simulink subsystem "LuT"  (R2019b)
settings: Solver=VariableStepAuto  StartTime=0.0  StopTime=10.0  RelTol=1e-3
undefined symbols (not defined in the file or in its folder): C1_lut, C2_lut, OCV_lut, R0_est, R0_lut, R1_lut, R2_lut
settings Model: Creator=PcElettronicaDynamis  LastModifiedBy=PcElettronicaDynamis

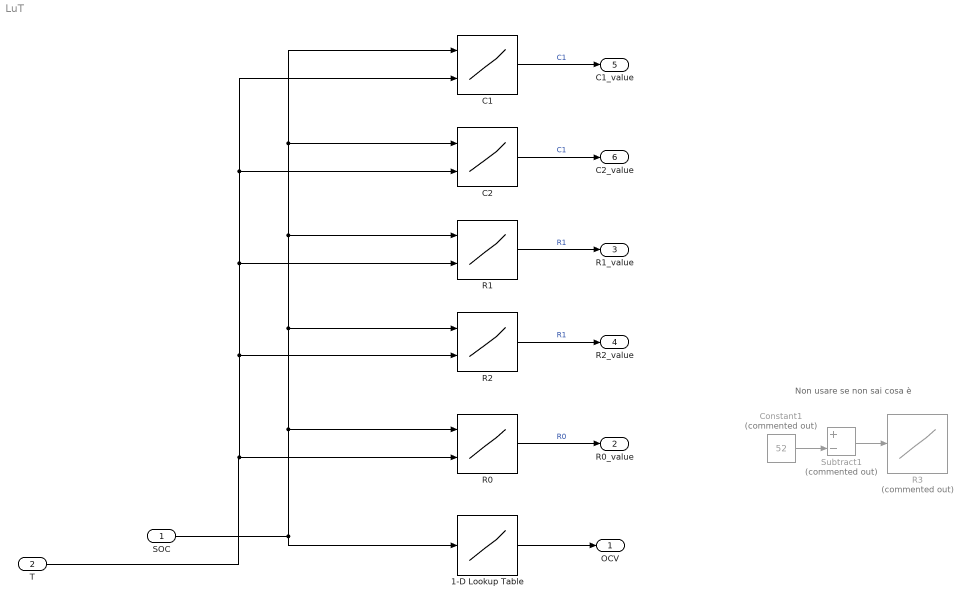
== system LuT ==
  note: Non usare se non sai cosa è
  SOC : Inport
  T : Inport  Port=2
  1-D Lookup Table : Lookup_n-D  NumberOfTableDimensions=1  BreakpointsForDimension1=[1:100]  BreakpointsForDimension2=[1:40]  BreakpointsForDimension1FirstPoint=0  BreakpointsForDimension1Spacing=10  Table=OCV_lut  InternalRulePriority=Speed  RndMeth=Simplest  InputSameDT=on
  C1 : Lookup_n-D  BreakpointsForDimension1=[1:100]  BreakpointsForDimension2=[1:40]  BreakpointsForDimension1FirstPoint=0  BreakpointsForDimension1Spacing=10  Table=C1_lut  InternalRulePriority=Speed  RndMeth=Simplest  InputSameDT=on
  C2 : Lookup_n-D  BreakpointsForDimension1=[1:100]  BreakpointsForDimension2=[1:40]  BreakpointsForDimension1FirstPoint=0  BreakpointsForDimension1Spacing=10  Table=C2_lut  InternalRulePriority=Speed  RndMeth=Simplest  InputSameDT=on
  Constant1 : Constant  Commented=on  Value=52
  R0 : Lookup_n-D  BreakpointsForDimension1=[1:100]  BreakpointsForDimension2=[1:40]  BreakpointsForDimension1FirstPoint=0  BreakpointsForDimension1Spacing=10  Table=R0_lut  InternalRulePriority=Speed  RndMeth=Simplest  InputSameDT=on
  R1 : Lookup_n-D  BreakpointsForDimension1=[1:100]  BreakpointsForDimension2=[1:40]  BreakpointsForDimension1FirstPoint=0  BreakpointsForDimension1Spacing=10  Table=R1_lut  InternalRulePriority=Speed  RndMeth=Simplest  InputSameDT=on
  R2 : Lookup_n-D  BreakpointsForDimension1=[1:100]  BreakpointsForDimension2=[1:40]  BreakpointsForDimension1FirstPoint=0  BreakpointsForDimension1Spacing=10  Table=R2_lut  InternalRulePriority=Speed  RndMeth=Simplest  InputSameDT=on
  R3 : Lookup_n-D  Commented=on  NumberOfTableDimensions=1  BreakpointsForDimension1=[1:32]  BreakpointsForDimension2=[1:40]  BreakpointsForDimension1FirstPoint=0  BreakpointsForDimension1Spacing=10  Table=R0_est  InternalRulePriority=Speed  RndMeth=Simplest  InputSameDT=on
  Subtract1 : Sum  Commented=on  Inputs=+-
  OCV : Outport
  R0_value : Outport  Port=2
  R1_value : Outport  Port=3
  R2_value : Outport  Port=4
  C1_value : Outport  Port=5
  C2_value : Outport  Port=6
  wires:
  C1/1 -> C1_value/1  "C1"
  R1/1 -> R1_value/1  "R1"
  R2/1 -> R2_value/1  "R1"
  C2/1 -> C2_value/1  "C1"
  T/1 -> R0/2, C2/2, C1/2, R1/2, R2/2
  SOC/1 -> 1-D Lookup Table/1, R0/1, R2/1, R1/1, C2/1, C1/1
  R0/1 -> R0_value/1  "R0"
  1-D Lookup Table/1 -> OCV/1
  Constant1/1 -> Subtract1/2
  Subtract1/1 -> R3/1
